simulink model "Phase4_Model_Reduced_students"  (R2023b)
settings: Solver=ode4  StartTime=0.0  StopTime=5  FixedStep=Ts  RelTol=1e-3
values from neighbouring files (symbols this model uses):
  Kf = Kc * T_1    [Task2_P4.m]    (also in linearized_model_students.m; task1_P4.m; task1_p4.m; task2_P4.m)
  Ph = [0.0322261797598 0.0141739364517 0.0605899881507 0.00105505375597 1.7477329169 0.0147577847461]    [ph.mat]
  q10 = 0    [Task2_P4.m]    (also in linearized_model_students.m; task1_P4.m; task1_p4.m; task2_P4.m)
  q20 = pi    (= 3.14159265359)    [Task2_P4.m]    (also in linearized_model_students.m; task1_P4.m; task1_p4.m; task2_P4.m)
  X0 = [0; 0.95*pi; 0; 0]    [Task2_P4.m]    (also in linearized_model_students.m; task1_P4.m; task1_p4.m; task2_P4.m)
settings Model: Creator=shahin  LastModifiedBy=shahin
settings DataIOCC: ReturnWorkspaceOutputs=off
settings OptimizationCC: ReuseModelBlockBuffer=off

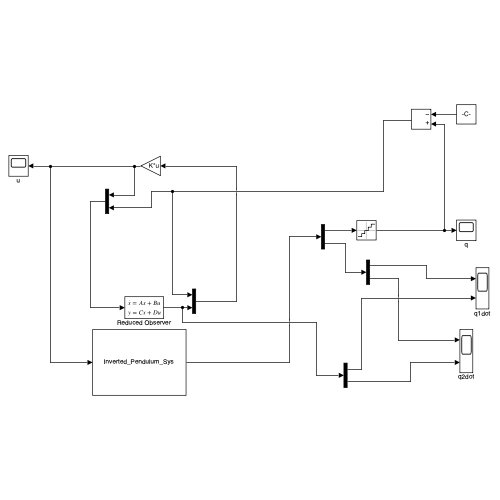
[thumbnail: Simulink's stored preview of the top-level diagram]
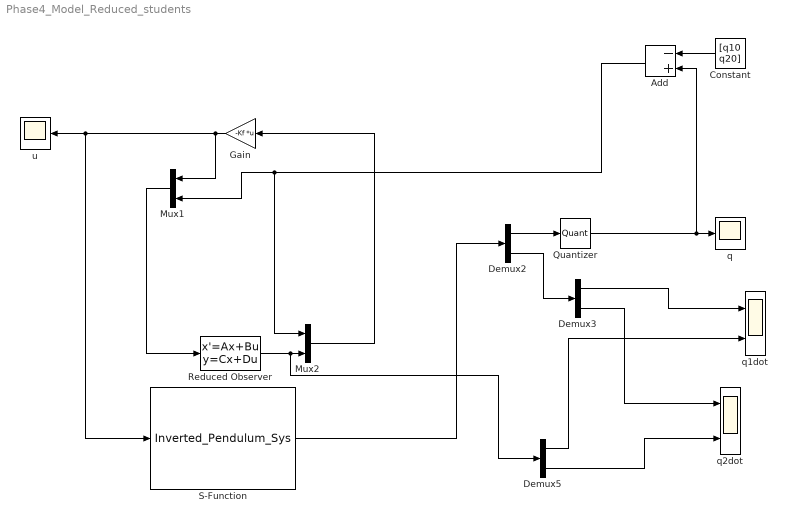
== system Phase4_Model_Reduced_students ==
  Add : Sum  Inputs=-+
  Constant : Constant  Value="[q10  q20]"
  Demux2 : Demux  Outputs=2
  Demux3 : Demux  Outputs=2
  Demux5 : Demux  Outputs=2
  Gain : Gain  Gain=-Kf  Multiplication=Matrix(K*u)
  Mux1 : Mux  Inputs=2
  Mux2 : Mux  Inputs=2
  Quantizer : Quantizer  QuantizationInterval="[2*pi/2048  2*pi/2048]"
  Reduced Observer : StateSpace  A=[]  C=[]  InitialCondition=[]
  S-Function : S-Function  FunctionName=Inverted_Pendulum_Sys  Parameters=X0,Ph  SFunctionDeploymentMode=off  EnableBusSupport=off
  q : Scope
  q1dot : Scope  NumInputPorts=2
  q2dot : Scope  NumInputPorts=2
  u : Scope
  wires:
  Demux2/1 -> Quantizer/1
  S-Function/1 -> Demux2/1
  Add/1 -> Mux2/1, Mux1/2
  Quantizer/1 -> Add/2, q/1
  Constant/1 -> Add/1
  Mux1/1 -> Reduced Observer/1
  Reduced Observer/1 -> Demux5/1, Mux2/2
  Mux2/1 -> Gain/1
  Demux2/2 -> Demux3/1
  Demux3/1 -> q1dot/1
  Demux3/2 -> q2dot/1
  Demux5/1 -> q1dot/2
  Gain/1 -> Mux1/1, S-Function/1, u/1
  Demux5/2 -> q2dot/2
